simulink model "RBG_einMassenmodell_Verifikation_Validierung"  (Simulink 8.3)
settings: Solver=ode45  StartTime=0.0  StopTime=15  MaxStep=0.02  RelTol=1e-3
libraries: simulink x2
settings Model: Creator=beck  LastModifiedBy=om8800
settings OptimizationCC: ExpressionDepthLimit=2147483647  InitFltsAndDblsToZero=on
settings DebuggingCC: SaveWithParameterizedLinksMsg=none  SignalResolutionControl=TryResolveAllWithWarning  FcnCallInpInsideContextMsg=EnableAllAsWarning  StrictBusMsg=Warning
settings RTWCC: IncludeERTFirstTime=on
settings GRTTargetCC: TargetFcnLib=ansi_tfl_tmw.mat

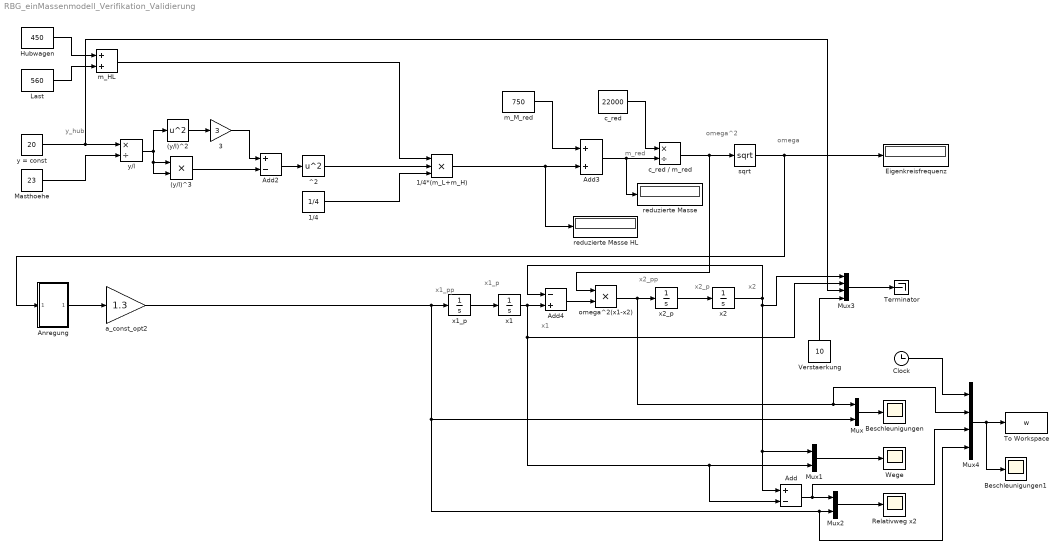
== system RBG_einMassenmodell_Verifikation_Validierung ==
  note: y_hub
  note: m_red
  note: omega^2
  note: x1_pp
  note: x2_pp
  note: x2_p
  note: x1_p
  note: omega
  note: x2
  note: x1
  (y/l)^2 : Math  Operator=square  SaturateOnIntegerOverflow=on
  (y/l)^3 : Product  RndMeth=Zero
  1/4 : Constant  Value=1/4
  1/4*(m_L+m_H) : Product  Inputs=3  RndMeth=Zero
  3 : Gain  Gain=3
  Add : Sum  Inputs=+-
  Add2 : Sum  Inputs=+-
  Add3 : Sum
  Add4 : Sum  Inputs=-+
  Anregung : Subsystem
  Beschleunigungen : Scope
      settings: YMin=-2  YMax=1.75  SaveName=ScopeData4
  Beschleunigungen1 : Scope
      settings: YMin=-0.5  YMax=3  SaveName=ScopeData7
  Clock : Clock
  Eigenkreisfrequenz : Display
  Hubwagen : Constant  Value=450
  Last : Constant  Value=560
  Masthoehe : Constant  Value=23
  Mux : Mux  Inputs=2
  Mux1 : Mux  Inputs=2
  Mux2 : Mux  Inputs=2
  Mux3 : Mux
  Mux4 : Mux
  Relativweg x2 : Scope
      settings: TimeRange=20  YMin=-2  YMax=2  SaveName=ScopeData6
  Terminator : Terminator
  To Workspace : ToWorkspace  VariableName=w  SampleTime=-1
  Verstaerkung : Constant  Value=10
  Wege : Scope
      settings: YMin=0  YMax=22
  ^2 : Math  Operator=square  SaturateOnIntegerOverflow=on
  a_const_opt2 : Gain  Gain=1.3
  c_red : Constant  Value=22000
  c_red / m_red : Product  Inputs=*/  RndMeth=Zero
  m_HL : Sum
  m_M_red : Constant  Value=750
  omega^2(x1-x2) : Product  RndMeth=Zero
  reduzierte Masse : Display
      settings: Decimation=2
  reduzierte Masse HL : Display
      settings: Decimation=2
  sqrt : Math  Operator=sqrt  SaturateOnIntegerOverflow=on
  x1 : Integrator
  x1_p : Integrator
  x2 : Integrator
  x2_p : Integrator
  y = const : Constant  Value=20
  y/l : Product  Inputs=*/  RndMeth=Zero
  wires:
  y = const/1 -> y/l/1, Mux3/3
  Mux/1 -> Beschleunigungen/1
  Mux1/1 -> Wege/1
  Masthoehe/1 -> y/l/2
  (y/l)^2/1 -> 3/1
  3/1 -> Add2/1
  (y/l)^3/1 -> Add2/2
  y/l/1 -> (y/l)^3/2, (y/l)^3/1, (y/l)^2/1
  c_red/1 -> c_red / m_red/1
  c_red / m_red/1 -> sqrt/1, omega^2(x1-x2)/1
  Add3/1 -> reduzierte Masse/1, c_red / m_red/2
  sqrt/1 -> Eigenkreisfrequenz/1, Anregung/1(In1)
  omega^2(x1-x2)/1 -> x2_p/1, Mux/1, Mux4/2
  x2_p/1 -> x2/1
  x1_p/1 -> x1/1
  Add4/1 -> omega^2(x1-x2)/2
  x1/1 -> Add4/2, Mux1/2, Add/2, Mux3/2
  x2/1 -> Add4/1, Add/1, Mux1/1, Mux3/1
  Verstaerkung/1 -> Mux3/4
  Add2/1 -> ^2/1
  m_M_red/1 -> Add3/1
  Mux2/1 -> Relativweg x2/1
  Add/1 -> Mux2/1, Mux4/3
  Last/1 -> m_HL/2
  Hubwagen/1 -> m_HL/1
  1/4*(m_L+m_H)/1 -> Add3/2, reduzierte Masse HL/1
  ^2/1 -> 1/4*(m_L+m_H)/2
  m_HL/1 -> 1/4*(m_L+m_H)/1
  1/4/1 -> 1/4*(m_L+m_H)/3
  a_const_opt2/1 -> x1_p/1, Mux/2, Mux2/2, Mux4/4
  Anregung/1(Out1) -> a_const_opt2/1
  Clock/1 -> Mux4/1
  Mux4/1 -> To Workspace/1, Beschleunigungen1/1
  Mux3/1 -> Terminator/1

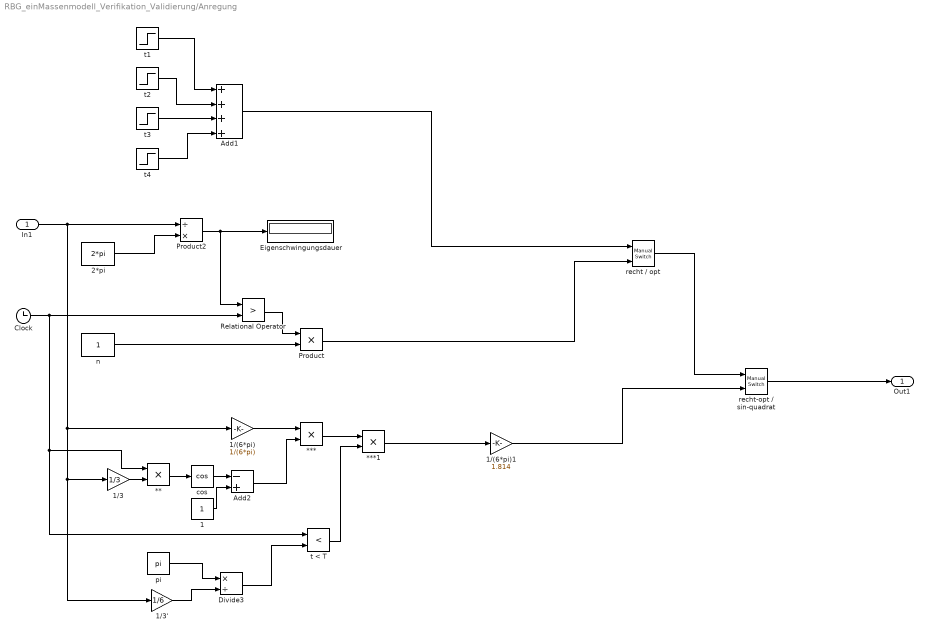
== system RBG_einMassenmodell_Verifikation_Validierung/Anregung ==
  In1 : Inport
  ** : Product  RndMeth=Zero
  *** : Product  RndMeth=Zero
  ***1 : Product  RndMeth=Zero
  1 : Constant
  1/(6*pi) : Gain  Gain=1/(6*pi)
  1/(6*pi)1 : Gain  Gain=1.814
  1/3 : Gain  Gain=1/3
  1/3' : Gain  Gain=1/6
  2*pi : Constant  Value=2*pi
  Add1 : Sum  Inputs=++++
  Add2 : Sum  Inputs=-+
  Clock : Clock
  Divide3 : Product  Inputs=*/
  Eigenschwingungsdauer : Display
  Product : Product  RndMeth=Zero
  Product2 : Product  Inputs=/*  RndMeth=Zero
  Relational Operator : RelationalOperator  Operator=>
  "cos " : Trigonometry  Operator=cos
  n : Constant
  pi : Constant  Value=pi
  recht / opt : simulink/Signal Routing/Manual Switch  sw=1  action=0  varsize=off
  recht-opt / sin-quadrat : simulink/Signal Routing/Manual Switch  sw=1  action=0  varsize=off
  t < T : RelationalOperator  Operator=<  OutDataTypeStr=boolean
  t1 : Step  Time=0  SampleTime=0
  t2 : Step  Time=2  After=-1  SampleTime=0
  t3 : Step  Time=8  After=-1  SampleTime=0
  t4 : Step  Time=10  SampleTime=0
  Out1 : Outport
  wires:
  2*pi/1 -> Product2/2
  t1/1 -> Add1/1
  t2/1 -> Add1/2
  Clock/1 -> Relational Operator/2, **/1, t < T/1
  n/1 -> Product/2
  t3/1 -> Add1/3
  t4/1 -> Add1/4
  Product2/1 -> Eigenschwingungsdauer/1, Relational Operator/1
  Relational Operator/1 -> Product/1
  Product/1 -> recht / opt/2
  In1/1 -> Product2/1, 1/(6*pi)/1, 1/3/1, 1/3'/1
  1/3/1 -> **/2
  **/1 -> "cos "/1
  "cos "/1 -> Add2/1
  1/1 -> Add2/2
  1/(6*pi)/1 -> ***/1
  Add2/1 -> ***/2
  ***/1 -> ***1/1
  pi/1 -> Divide3/1
  Divide3/1 -> t < T/2
  t < T/1 -> ***1/2
  recht-opt / sin-quadrat/1 -> Out1/1
  1/3'/1 -> Divide3/2
  ***1/1 -> 1/(6*pi)1/1
  1/(6*pi)1/1 -> recht-opt / sin-quadrat/2
  Add1/1 -> recht / opt/1
  recht / opt/1 -> recht-opt / sin-quadrat/1
